simulink model "ACCBase004_dist"  (Simulink 8.3)
settings: Solver=FixedStepDiscrete  StartTime=0.0  StopTime=10.0  FixedStep=0.1  RelTol=1e-3
model workspace (MAT data in the model file):
  pACC.Kp = 0.1
  pACC.minDist2Target = 50
  pACC.Ki = 0.0001
  pACC.KpDist = 1
  pACC.KiDist : numeric (value not decoded)
libraries: Lib_Controls x3
settings Model: Creator=swami  LastModifiedBy=swami
settings DataIOCC: SignalLoggingSaveFormat=Dataset
settings DebuggingCC: UnderspecifiedInitializationDetection=Simplified  StateNameClashWarn=none
settings GRTTargetCC: CombineOutputUpdateFcns=on  GRTInterface=off

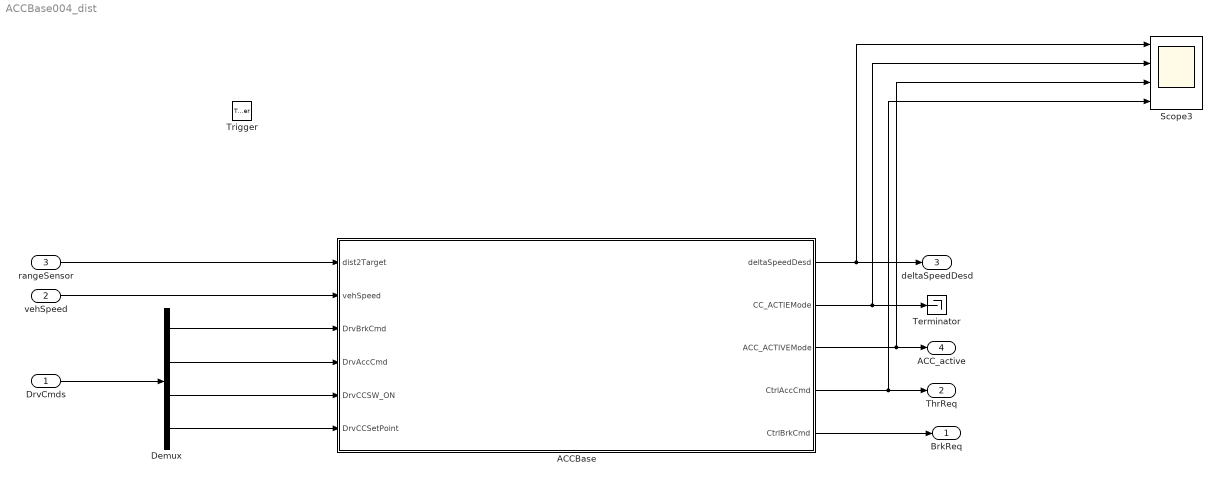
== system ACCBase004_dist ==
  DrvCmds : Inport  PortDimensions=4
  vehSpeed : Inport  Port=2
  rangeSensor : Inport  Port=3
  Trigger : TriggerPort  TriggerType=function-call  PortDimensions=1
  ACCBase : Subsystem  mask{minDist2Target=pACC.minDist2Target, ACCBuffer=pACC.minDist2Target*0.9, Kp=pACC.Kp, Ki=pACC.Ki, KpDist=pACC.KpDist, KiDist=pACC.KiDist}
  Demux : Demux
  Scope3 : Scope  NumInputPorts=4
      settings: TimeRange=50  YMin=-5~-5~-5~-5  YMax=5~5~5~5  SaveName=ScopeData4
  Terminator : Terminator
  BrkReq : Outport  PortDimensions=1
  ThrReq : Outport  Port=2  PortDimensions=1
  deltaSpeedDesd : Outport  Port=3  PortDimensions=1
  ACC_active : Outport  Port=4  PortDimensions=1
  wires:
  DrvCmds/1 -> Demux/1
  Demux/3 -> ACCBase/5(DrvCCSW_ON)
  Demux/4 -> ACCBase/6(DrvCCSetPoint)
  rangeSensor/1 -> ACCBase/1(dist2Target)
  vehSpeed/1 -> ACCBase/2(vehSpeed)
  ACCBase/3(ACC_ACTIVEMode) -> Scope3/3, ACC_active/1
  ACCBase/5(CtrlBrkCmd) -> BrkReq/1
  ACCBase/1(deltaSpeedDesd) -> Scope3/1, deltaSpeedDesd/1
  ACCBase/4(CtrlAccCmd) -> Scope3/4, ThrReq/1
  ACCBase/2(CC_ACTIEMode) -> Scope3/2, Terminator/1
  Demux/1 -> ACCBase/3(DrvBrkCmd)
  Demux/2 -> ACCBase/4(DrvAccCmd)

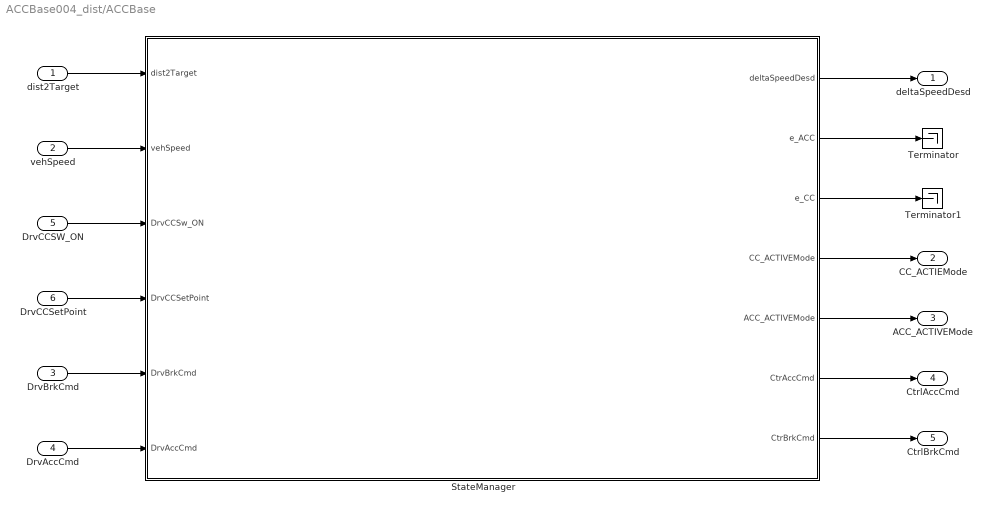
== system ACCBase004_dist/ACCBase ==
  dist2Target : Inport
  vehSpeed : Inport  Port=2
  DrvBrkCmd : Inport  Port=3
  DrvAccCmd : Inport  Port=4
  DrvCCSW_ON : Inport  Port=5
  DrvCCSetPoint : Inport  Port=6
  StateManager : Stateflow chart  TreatAsAtomicUnit=on
  Terminator : Terminator
  Terminator1 : Terminator
  deltaSpeedDesd : Outport
  CC_ACTIEMode : Outport  Port=2
  ACC_ACTIVEMode : Outport  Port=3
  CtrlAccCmd : Outport  Port=4
  CtrlBrkCmd : Outport  Port=5
  wires:
  DrvCCSetPoint/1 -> StateManager/4(DrvCCSetPoint)
  DrvAccCmd/1 -> StateManager/6(DrvAccCmd)
  DrvCCSW_ON/1 -> StateManager/3(DrvCCSw_ON)
  dist2Target/1 -> StateManager/1(dist2Target)
  StateManager/5(" ACC_ACTIVEMode") -> ACC_ACTIVEMode/1
  StateManager/1(deltaSpeedDesd) -> deltaSpeedDesd/1
  StateManager/4(" CC_ACTIVEMode") -> CC_ACTIEMode/1
  DrvBrkCmd/1 -> StateManager/5(DrvBrkCmd)
  vehSpeed/1 -> StateManager/2(vehSpeed)
  StateManager/6(CtrAccCmd) -> CtrlAccCmd/1
  StateManager/7(CtrBrkCmd) -> CtrlBrkCmd/1
  StateManager/2(e_ACC) -> Terminator/1
  StateManager/3(e_CC) -> Terminator1/1

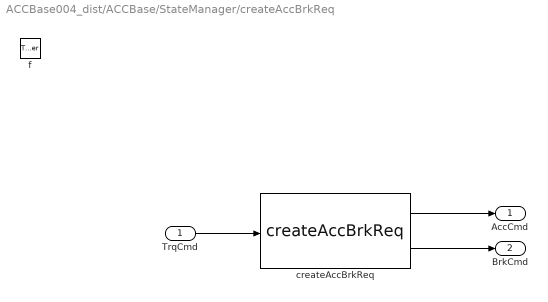
== system ACCBase004_dist/ACCBase/StateManager/createAccBrkReq ==
  TrqCmd : Inport  OutDataTypeStr=double  PortDimensions=1
  f : TriggerPort  TriggerType=function-call
      settings: CopyFcn=Stateflow.SLINSF.SimulinkMan.removeBlockPreDeleteFcn  PreDeleteFcn=Stateflow.SLINSF.SimulinkMan.unsafePredeleteFcn
  createAccBrkReq : Lib_Controls/createAccBrkReq
  AccCmd : Outport
  BrkCmd : Outport  Port=2
  wires:
  TrqCmd/1 -> createAccBrkReq/1
  createAccBrkReq/1 -> AccCmd/1
  createAccBrkReq/2 -> BrkCmd/1

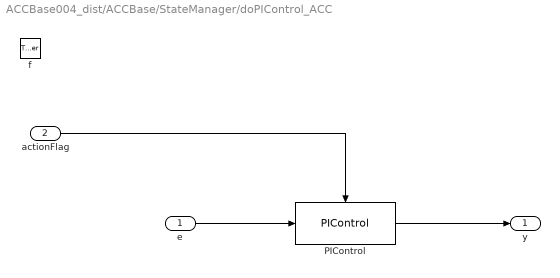
== system ACCBase004_dist/ACCBase/StateManager/doPIControl_ACC ==
  e : Inport  OutDataTypeStr=double  PortDimensions=1
  actionFlag : Inport  Port=2  OutDataTypeStr=double  PortDimensions=1
  f : TriggerPort  TriggerType=function-call
      settings: CopyFcn=Stateflow.SLINSF.SimulinkMan.removeBlockPreDeleteFcn  PreDeleteFcn=Stateflow.SLINSF.SimulinkMan.unsafePredeleteFcn
  PIControl : Lib_Controls/PIControl  Kp=KpDist  Ki=KiDist
  y : Outport
  wires:
  PIControl/1 -> y/1
  e/1 -> PIControl/1
  actionFlag/1 -> PIControl/Enable

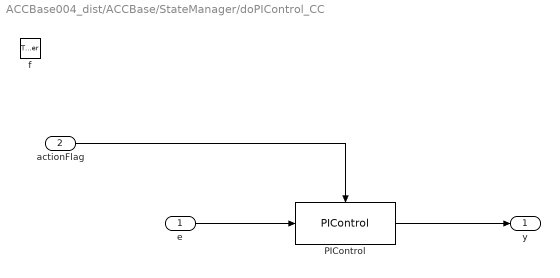
== system ACCBase004_dist/ACCBase/StateManager/doPIControl_CC ==
  e : Inport  OutDataTypeStr=double  PortDimensions=1
  actionFlag : Inport  Port=2  OutDataTypeStr=double  PortDimensions=1
  f : TriggerPort  TriggerType=function-call
      settings: CopyFcn=Stateflow.SLINSF.SimulinkMan.removeBlockPreDeleteFcn  PreDeleteFcn=Stateflow.SLINSF.SimulinkMan.unsafePredeleteFcn
  PIControl : Lib_Controls/PIControl  Kp=Kp  Ki=Ki
      link override Constant: Value=0
  y : Outport
  wires:
  PIControl/1 -> y/1
  e/1 -> PIControl/1
  actionFlag/1 -> PIControl/Enable

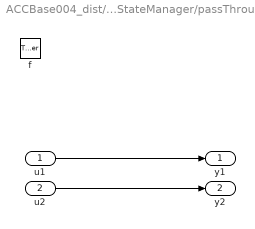
== system ACCBase004_dist/ACCBase/StateManager/passThrough ==
  u1 : Inport  OutDataTypeStr=double  PortDimensions=1
  u2 : Inport  Port=2  OutDataTypeStr=double  PortDimensions=1
  f : TriggerPort  TriggerType=function-call
      settings: CopyFcn=Stateflow.SLINSF.SimulinkMan.removeBlockPreDeleteFcn  PreDeleteFcn=Stateflow.SLINSF.SimulinkMan.unsafePredeleteFcn
  y1 : Outport
  y2 : Outport  Port=2
  wires:
  u1/1 -> y1/1
  u2/1 -> y2/1

== stateflow chart ACCBase/StateManager ==
  state CC_ACTIVE
    entry:
    deltaSpeedDesd = 0;
    e_CC = (DrvCCSetPoint + deltaSpeedDesd - vehSpeed);
    doPIControl_CC(e_CC,startAction);
    during:
    e_CC = (DrvCCSetPoint + deltaSpeedDesd - vehSpeed);
    [CtrAccCmd, CtrBrkCmd]  = createAccBrkReq(doPIControl_CC(e_CC,doAction));
    exit:
    [CtrAccCmd, CtrBrkCmd]  = createAccBrkReq(doPIControl_CC(e_CC,stopAction));
    state ACC_ACTIVE
      entry:
      e_ACC = dist2Target - minDist2Target;
      doPIControl_ACC(e_ACC,startAction);
      during:
      e_ACC = dist2Target - minDist2Target;
      deltaSpeedDesd = doPIControl_ACC(e_ACC,doAction);
    state ACC_INACTIVE
      entry:
      deltaSpeedDesd = 0;
    (default) -> ACC_INACTIVE
    ACC_ACTIVE -> ACC_INACTIVE [order 2] : [turn_ACC_OFF]
    ACC_ACTIVE -> ACC_INACTIVE [order 1] : [dist2Target>(minDist2Target + ACCBuffer)]
    ACC_INACTIVE -> ACC_ACTIVE : [dist2Target < minDist2Target]
    ACC_ACTIVE -> ACC_ACTIVE [order 3] : [deltaSpeedDesd > 0]
        |   {deltaSpeedDesd = 0;
        |    turn_ACC_OFF = true;}
  state CC_INACTIVE
    during:
    [CtrAccCmd, CtrBrkCmd] = passThrough(DrvAccCmd, DrvBrkCmd);
  state [y1,y2] = passThrough(u1,u2) [function]
  state y = doPIControl_CC(e,actionFlag) [function]
  state [AccCmd, BrkCmd] = createAccBrkReq(TrqCmd) [function]
  state y = doPIControl_ACC(e,actionFlag) [function]
  (default) -> CC_INACTIVE
  CC_ACTIVE -> CC_INACTIVE : [DrvCCSw_ON<0.5]
  CC_INACTIVE -> CC_ACTIVE : [DrvCCSw_ON>0.5]
  data: u1 function_input double size=1; u2 function_input double size=1; y1 function_output double; y2 function_output double; e function_input double size=1; y function_output double; actionFlag function_input double size=1; TrqCmd function_input double size=1; AccCmd function_output double; BrkCmd function_output double; e function_input double size=1; y function_output double; actionFlag function_input double size=1; minDist2Target parameter double; dist2Target input double; ACCBuffer parameter double; turn_ACC_OFF local double; vehSpeed input double; DrvCCSw_ON input double; deltaSpeedDesd output double; e_ACC output double; e_CC output double; CC_ACTIVEMode output boolean; ACC_ACTIVEMode output boolean; DrvCCSetPoint input double; DrvBrkCmd input double; DrvAccCmd input double; CtrAccCmd output double; CtrBrkCmd output double; stopAction constant double =0; doAction constant double =2; startAction constant double =1
